simulink model "BurstRxModel"  (R2026a)
settings: Solver=FixedStepDiscrete  StopTime=20000
libraries: dsphdlxfrm2 x1, simulink x1
settings Model: DataTypeOverride=Off  Creator=jiemingx  LastModifiedBy=jiemingx
settings OptimizationCC: ConditionallyExecuteInputs=off  InheritOutputTypeSmallerThanSingle=on
settings DebuggingCC: ArtificialAlgebraicLoopMsg=error  MergeDetectMultiDrivingBlocksExec=error  SingleTaskRateTransMsg=error
settings HardwareCC: ProdHWDeviceType=ASIC/FPGA->ASIC/FPGA  TargetBitPerLong=64.0  TargetBitPerPointer=64.0  TargetBitPerSizeT=64.0  TargetBitPerPtrDiffT=64.0  TargetLongLongMode=on  TargetIntDivRoundTo=Zero  TargetEndianess=LittleEndian  TargetWordSize=64.0  TargetHWDeviceType=Custom Processor->MATLAB Host Computer  ProdEqTarget=off
settings ModelReferenceCC: PropagateSignalLabelsOutOfModel=on

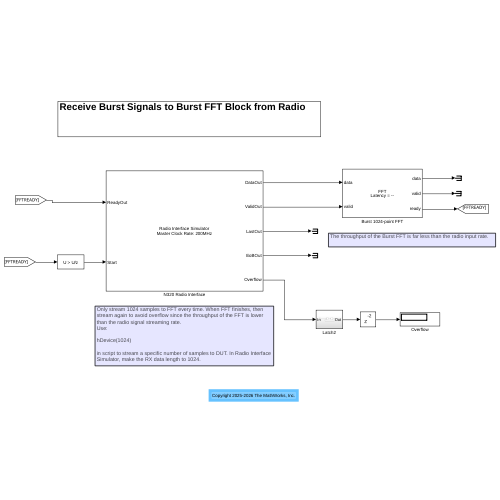
[thumbnail: Simulink's stored preview of the top-level diagram]
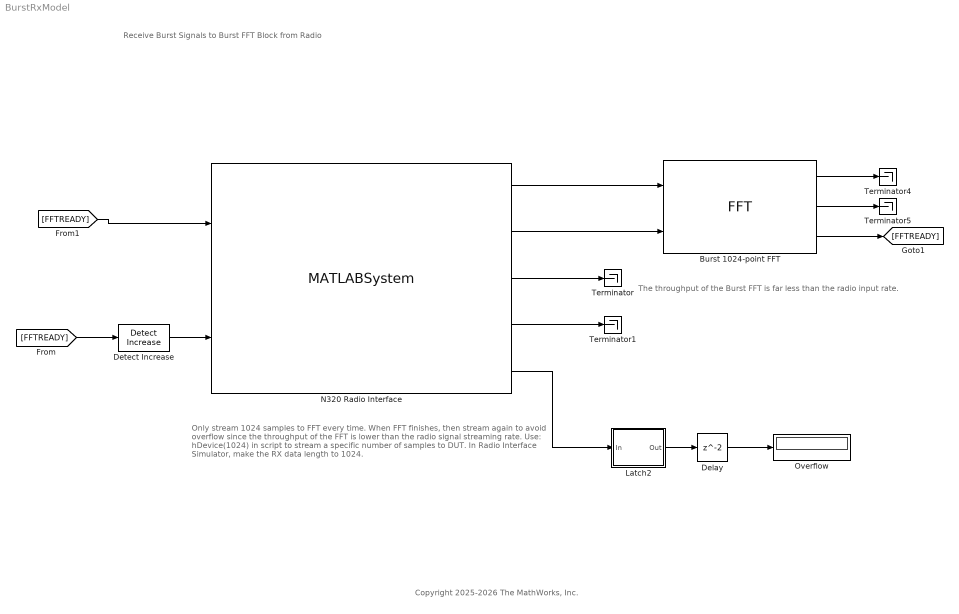
== system BurstRxModel ==
  note: The throughput of the Burst FFT is far less than the radio input rate.
  note: Receive Burst Signals to Burst FFT Block from Radio
  note: Only stream 1024 samples to FFT every time. When FFT finishes, then
      | stream again to avoid overflow since the throughput of the FFT is lower
      | than the radio signal streaming rate.
      | Use:
      |
      | hDevice(1024)
      |
      | in script to stream a specific number of samples to DUT. In Radio Interface
      | Simulator, make the RX data length to 1024.
  note: Copyright 2025-2026 The MathWorks, Inc.
  Burst 1024-point FFT : dsphdlxfrm2/FFT  Architecture=Burst Radix 2  FFTLengthSource=Property  FFTLength=1024  FFTLengthMax=1024  ComplexMultiplication=Use 4 multipliers and 2 adders  BitReversedOutput=on  BitReversedInput=off  Normalize=off  SimulateUsing=Code generation  RoundingMethod=Floor  ResetInputPort=off  StartOutputPort=off  EndOutputPort=off
  Delay : Delay  SampleTime=1
  Detect Increase : simulink/Logic and Bit Operations/Detect Increase  vinit=0.0  OutDataTypeStr=boolean
      settings: LibrarySourceBlock=|
      | hdlsllib/Logic and Bit
      | Operations/Detect
      | Increase
  Latch2 : Subsystem
  N320 Radio Interface : MATLABSystem  System=RadioInterfaceSim  Device=N320  TXRX=RX  ClockSource=Radio  SampleRate=200e6  DUTClockRate=61.44e6  InputDataSource=int16(rand(1,5024))  SimulateUsing=Code generation  ClockUncertainty=off  Uncertainty=0  Jitter=0
      mask Type: RadioInterfaceSim
  Overflow : Display
  Terminator{,1,4..5} (4 alike) : Terminator
  wires:
  N320 Radio Interface/5 -> Latch2/1(In)
  Latch2/1(Out) -> Delay/1
  Burst 1024-point FFT/2 -> Terminator5/1
  Burst 1024-point FFT/1 -> Terminator4/1
  Burst 1024-point FFT/3 -> [FFTREADY]
  [FFTREADY] -> Detect Increase/1
  Detect Increase/1 -> N320 Radio Interface/2
  N320 Radio Interface/1 -> Burst 1024-point FFT/1
  N320 Radio Interface/2 -> Burst 1024-point FFT/2
  [FFTREADY] -> N320 Radio Interface/1
  N320 Radio Interface/3 -> Terminator/1
  N320 Radio Interface/4 -> Terminator1/1
  Delay/1 -> Overflow/1

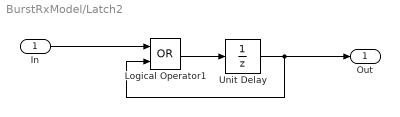
== system BurstRxModel/Latch2 ==
  In : Inport
  Logical Operator1 : Logic  Operator=OR  AllPortsSameDT=off  OutDataTypeStr=boolean
  Unit Delay : UnitDelay  SampleTime=-1
  Out : Outport
  wires:
  Unit Delay/1 -> Out/1, Logical Operator1/2
  In/1 -> Logical Operator1/1
  Logical Operator1/1 -> Unit Delay/1
